simulink model "Transitions8"  (R2020a)
settings: Solver=VariableStepAuto  StartTime=0.0  StopTime=0.5  RelTol=1e-3
settings Model: Creator=BEAR  LastModifiedBy=bzhan
settings DataIOCC: ReturnWorkspaceOutputs=off
settings DebuggingCC: ArithmeticOperatorsInVariantConditions=warning
settings SFSimCC: SimUseLocalCustomCode=off  CustomCodeUndefinedFunction=UseInterfaceOnly
settings RTWCC: RTWUseLocalCustomCode=off

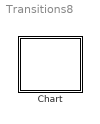
== system Transitions8 ==
  Chart : Stateflow chart  TreatAsAtomicUnit=on

== stateflow chart Transitions8/Chart ==
  settings: updateMethod=DISCRETE  sampleTime=0.1
  state S
    en: f("enS")
    du: f("duS")
    S -> S [order 1] : [x<3]{f("ca1");x=x+1;}
    S -> S [order 2] : {f("ca2");x=x+1;}
  state T
    en: f("enT")
  (default) -> S : {x=1;}
  S -> T [order 1] : [x>=5]
  data: s function_input; x local
  function f(s):
    | function f(s)
    |   fprintf(s+"\n");
